simulink model "jacobi"  (R2021a)
settings: Solver=FixedStepDiscrete  StartTime=0.0  StopTime=10  FixedStep=1  RelTol=1e-3
libraries: dspmtrx3 x4, dspinverses x1, simulink x1
settings Model: Creator=manur  LastModifiedBy=manur

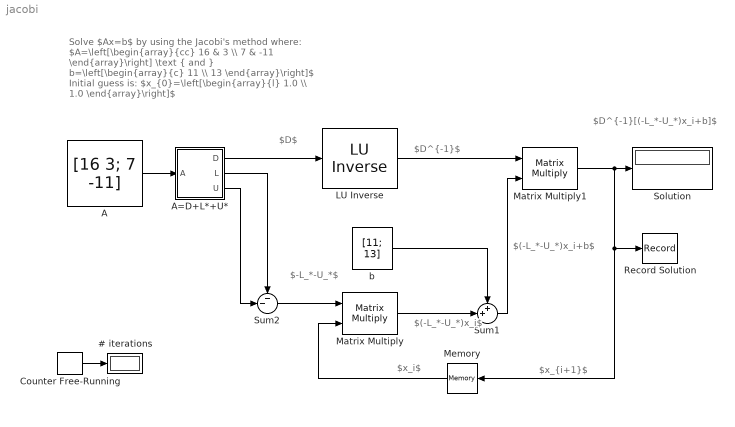
== system jacobi ==
  note: Solve $Ax=b$ by using the Jacobi's method where:
      | $A=\left[\begin{array}{cc} 16 & 3 \\ 7 & -11 \end{array}\right] \text { and } b=\left[\begin{array}{c} 11 \\ 13 \end{array}\right]$
      | Initial guess is:
      | $x_{0}=\left[\begin{array}{l} 1.0 \\ 1.0 \end{array}\right]$
  note: $D$
  note: $D^{-1}$
  note: $D^{-1}[(-L_*-U_*)x_i+b]$
  note: $x_i$
  note: $x_{i+1}$
  note: $-L_*-U_*$
  note: $(-L_*-U_*)x_i$
  note: $(-L_*-U_*)x_i+b$
  " LU Inverse" : dspinverses/ LU Inverse
  # iterations : Display
  A : Constant  Value=[16 3; 7 -11]
  A=D+L*+U* : Subsystem
      mask Display: image('$imagefile'); % Use "Edit Image" on toolstrip to change.
  Counter Free-Running : simulink/Sources/Counter Free-Running  NumBits=16  tsamp=-1
  Matrix Multiply : Product  Multiplication=Matrix(*)
  Matrix Multiply1 : Product  Multiplication=Matrix(*)
  Memory : Memory  InitialCondition=[1; 1]
  Record Solution : Record  FileSettingsInternal="{\"entries\":[{\"content\":{\"excelSettings\":{\"content\":{},\"type\":\"Streamout.ExcelSettings\"}},\"type\":\"Streamout.FileSettingStorage\",\"uuid\":\"fdd928e6-da05-4ea5-9392-d2ea8f7b474c\"}],\"packageUris\":[\"http://schema.mathworks.com/mf0/streamout_blocks/R2020a\"],\"version\":\"1.0\"}"  Layout=[1 1]  SignalsInternal="{\"entries\":[{\"content\":{\"signals\":[{\"content\":{\"blockPath\":[\"jacobi/Record\"],\"channel\":[],\"dimensions\":[2,1],\"domain\":\"jacobi/record\",\"hasChildren\":true,\"lineColor\":\"#fe330a\",\"plots\":[],\"port\":1,\"sid\":[\"\"],\"signalID\":235,\"signalName\":\"Matrix Multiply1\"},\"type\":\"RecordBlkView.Signal\",\"uuid\":\"3de9a350-0334-445e-b397-e6b2fc6ecd40\"},{\"content\":{\"blockPath\":[\"jacobi/Record\"],\"channel\":[1,1],\"dimensions\":[2,1],\"domain\":\"jacobi/record\",\"lineColor\":\"#7e2f8e\",\"parentID\":235,\"plots\":[1],\"port\":1,\"sid\":[\"\"],\"signalID\":236,\"signalName\":\"Matrix Multiply1\"},\"type\":\"RecordBlkView.Signal\",\"uuid\":\"c3de3b8d-272d-4ee7-8c88-4731baacc764\"},{\"content\":{\"blockPath\":[\"jacobi/Record\"],\"channel\":[2,1],\"dimensions\":[2,1],\"domain\":\"jacobi/record\",\"lineColor\":\"#a2142f\",\"parentID\":235,\"plots\":[],\"port\":1,\"sid\":[\"\"],\"signalID\":250,\"signalName\":\"Matrix Multiply1\"},\"type\":\"RecordBlkView.Signal\",\"uuid\":\"b403840d-4891-4daa-b62e-e2558c0d09b7\"}]},\"type\":\"RecordBlkView.InputSignals\",\"uuid\":\"1cda7f8f-2a05-4beb-adc3-2e8851fd8335\"}],\"packageUris\":[\"http://schema.mathworks.com/mf0/streamout_blocks/R2020a\"],\"version\":\"1.0\"}"  VisualizationBindings="{\"sparklinesplugin\":{\"info\":[{\"bindingParametersList\":[],\"subplotID\":1}]}}"
  Solution : Display
  Sum1 : Sum  Inputs=++|
  Sum2 : Sum  Inputs=--|
  b : Constant  Value=[11; 13]  VectorParams1D=off
  wires:
  Counter Free-Running/1 -> # iterations/1
  A/1 -> A=D+L*+U*/1(A)
  " LU Inverse"/1 -> Matrix Multiply1/1
  Matrix Multiply1/1 -> Memory/1, Record Solution/1, Solution/1
  Memory/1 -> Matrix Multiply/2
  Sum2/1 -> Matrix Multiply/1
  Matrix Multiply/1 -> Sum1/2
  b/1 -> Sum1/1
  Sum1/1 -> Matrix Multiply1/2
  A=D+L*+U*/1(D) -> " LU Inverse"/1
  A=D+L*+U*/2(L) -> Sum2/1
  A=D+L*+U*/3(U) -> Sum2/2

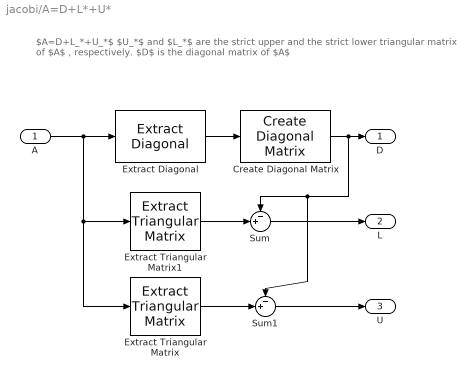
== system jacobi/A=D+L*+U* ==
  note: $A=D+L_*+U_*$
      | $U_*$ and $L_*$ are the strict upper and the strict lower triangular matrix of $A$ , respectively.
      | $D$ is the diagonal matrix of $A$
  A : Inport
  Create Diagonal Matrix : dspmtrx3/Create Diagonal Matrix
      settings: SourceProductBaseCode=DS
  Extract Diagonal : dspmtrx3/Extract Diagonal
      settings: SourceProductBaseCode=DS
  Extract Triangular Matrix : dspmtrx3/Extract Triangular Matrix  fcn=Upper  SimulateUsing=Code generation
      settings: SourceProductBaseCode=DS
  Extract Triangular Matrix1 : dspmtrx3/Extract Triangular Matrix  fcn=Lower  SimulateUsing=Code generation
      settings: SourceProductBaseCode=DS
  Sum : Sum  Inputs=-+|
  Sum1 : Sum  Inputs=-+|
  D : Outport
  L : Outport  Port=2
  U : Outport  Port=3
  wires:
  Extract Diagonal/1 -> Create Diagonal Matrix/1
  A/1 -> Extract Diagonal/1, Extract Triangular Matrix1/1, Extract Triangular Matrix/1
  Create Diagonal Matrix/1 -> D/1, Sum1/1, Sum/1
  Sum/1 -> L/1
  Extract Triangular Matrix1/1 -> Sum/2
  Extract Triangular Matrix/1 -> Sum1/2
  Sum1/1 -> U/1
